simulink model "System_Design_Quadrocopter"  (Simulink 7.4)
settings: Solver=ode45  StartTime=0.0  StopTime=10.0  RelTol=1e-3
settings Model: Creator=roczit00  LastModifiedBy=roczit00

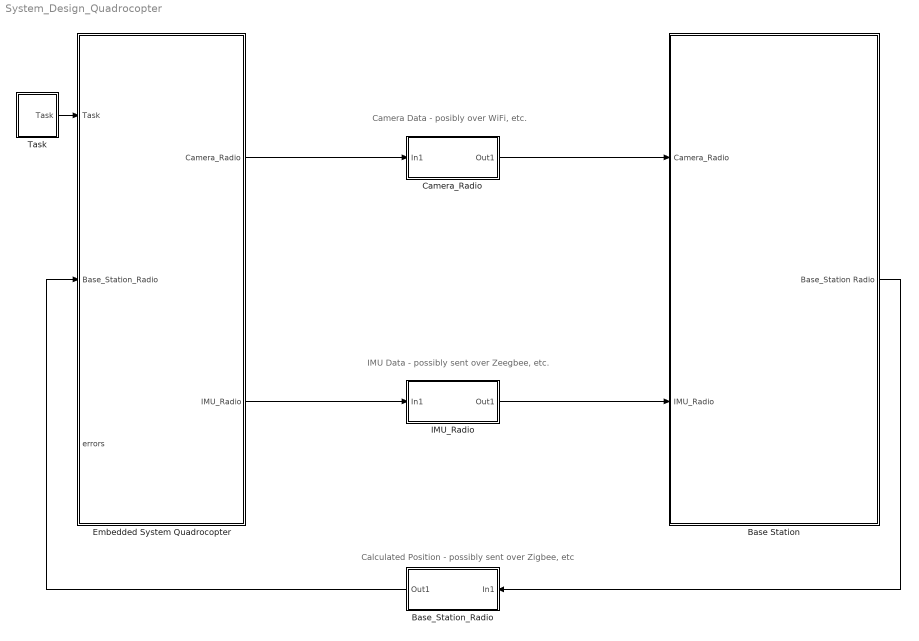
== system System_Design_Quadrocopter ==
  note: IMU Data - possibly sent over Zeegbee, etc.
  note: Calculated Position - possibly sent over Zigbee, etc
  note: Camera Data - posibly over WiFi, etc.
  Base Station : Subsystem
  Base_Station_Radio : Subsystem
  Camera_Radio : Subsystem
  Embedded System Quadrocopter : Subsystem
  IMU_Radio : Subsystem
  Task : Subsystem
  wires:
  Embedded System Quadrocopter/1(Camera_Radio) -> Camera_Radio/1(In1)
  Base Station/1(Base_Station Radio) -> Base_Station_Radio/1(In1)
  Base_Station_Radio/1(Out1) -> Embedded System Quadrocopter/2(Base_Station_Radio)
  Embedded System Quadrocopter/2(IMU_Radio) -> IMU_Radio/1(In1)
  IMU_Radio/1(Out1) -> Base Station/2(IMU_Radio)
  Camera_Radio/1(Out1) -> Base Station/1(Camera_Radio)
  Task/1(Task) -> Embedded System Quadrocopter/1(Task)

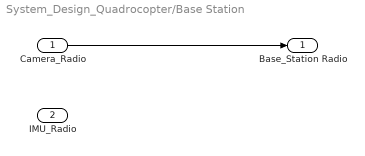
== system System_Design_Quadrocopter/Base Station ==
  Camera_Radio : Inport  OutDataType=fixdt(1, 16)  OutScaling=2^0
  IMU_Radio : Inport  Port=2  OutDataType=fixdt(1, 16)  OutScaling=2^0
  Base_Station Radio : Outport  OutDataType=fixdt(1, 16)  OutScaling=2^0
  wires:
  Camera_Radio/1 -> Base_Station Radio/1

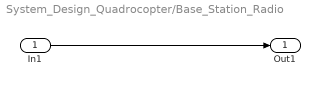
== system System_Design_Quadrocopter/Base_Station_Radio ==
  In1 : Inport  OutDataType=fixdt(1, 16)  OutScaling=2^0
  Out1 : Outport  OutDataType=fixdt(1, 16)  OutScaling=2^0
  wires:
  In1/1 -> Out1/1

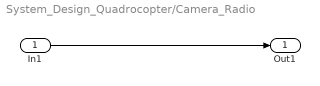
== system System_Design_Quadrocopter/Camera_Radio ==
  In1 : Inport  OutDataType=fixdt(1, 16)  OutScaling=2^0
  Out1 : Outport  OutDataType=fixdt(1, 16)  OutScaling=2^0
  wires:
  In1/1 -> Out1/1

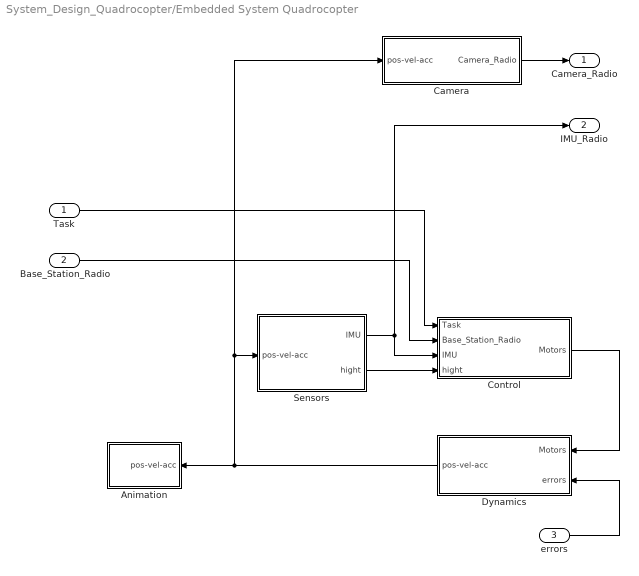
== system System_Design_Quadrocopter/Embedded System Quadrocopter ==
  Task : Inport  OutDataType=fixdt(1, 16)  OutScaling=2^0
  Base_Station_Radio : Inport  Port=2  OutDataType=fixdt(1, 16)  OutScaling=2^0
  errors : Inport  Port=3  OutDataType=fixdt(1, 16)  OutScaling=2^0
  Animation : Subsystem
  Camera : Subsystem
  Control : Subsystem
  Dynamics : Subsystem
  Sensors : Subsystem
  Camera_Radio : Outport  OutDataType=fixdt(1, 16)  OutScaling=2^0
  IMU_Radio : Outport  Port=2  OutDataType=fixdt(1, 16)  OutScaling=2^0
  wires:
  Sensors/1(IMU) -> Control/3(IMU), IMU_Radio/1
  Sensors/2(hight) -> Control/4(hight)
  errors/1 -> Dynamics/2(errors)
  Control/1(Motors) -> Dynamics/1(Motors)
  Dynamics/1(pos-vel-acc) -> Animation/1(pos-vel-acc), Sensors/1(pos-vel-acc), Camera/1(pos-vel-acc)
  Camera/1(Camera_Radio) -> Camera_Radio/1
  Base_Station_Radio/1 -> Control/2(Base_Station_Radio)
  Task/1 -> Control/1(Task)

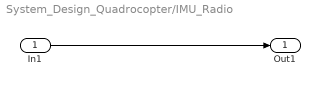
== system System_Design_Quadrocopter/IMU_Radio ==
  In1 : Inport  OutDataType=fixdt(1, 16)  OutScaling=2^0
  Out1 : Outport  OutDataType=fixdt(1, 16)  OutScaling=2^0
  wires:
  In1/1 -> Out1/1

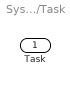
== system System_Design_Quadrocopter/Task ==
  Task : Outport  OutDataType=fixdt(1, 16)  OutScaling=2^0

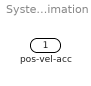
== system System_Design_Quadrocopter/Embedded System Quadrocopter/Animation ==
  pos-vel-acc : Inport  OutDataType=fixdt(1, 16)  OutScaling=2^0

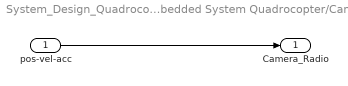
== system System_Design_Quadrocopter/Embedded System Quadrocopter/Camera ==
  pos-vel-acc : Inport  OutDataType=fixdt(1, 16)  OutScaling=2^0
  Camera_Radio : Outport  OutDataType=fixdt(1, 16)  OutScaling=2^0
  wires:
  pos-vel-acc/1 -> Camera_Radio/1

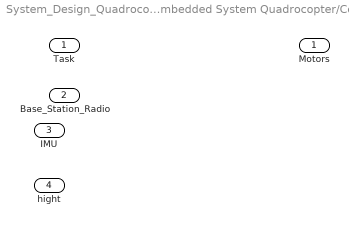
== system System_Design_Quadrocopter/Embedded System Quadrocopter/Control ==
  Task : Inport  OutDataType=fixdt(1, 16)  OutScaling=2^0
  Base_Station_Radio : Inport  Port=2  OutDataType=fixdt(1, 16)  OutScaling=2^0
  IMU : Inport  Port=3  OutDataType=fixdt(1, 16)  OutScaling=2^0
  hight : Inport  Port=4  OutDataType=fixdt(1, 16)  OutScaling=2^0
  Motors : Outport  OutDataType=fixdt(1, 16)  OutScaling=2^0

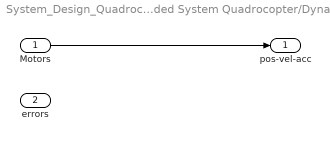
== system System_Design_Quadrocopter/Embedded System Quadrocopter/Dynamics ==
  Motors : Inport  OutDataType=fixdt(1, 16)  OutScaling=2^0
  errors : Inport  Port=2  OutDataType=fixdt(1, 16)  OutScaling=2^0
  pos-vel-acc : Outport  OutDataType=fixdt(1, 16)  OutScaling=2^0
  wires:
  Motors/1 -> pos-vel-acc/1

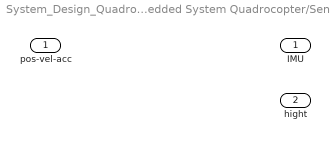
== system System_Design_Quadrocopter/Embedded System Quadrocopter/Sensors ==
  pos-vel-acc : Inport  OutDataType=fixdt(1, 16)  OutScaling=2^0
  IMU : Outport  OutDataType=fixdt(1, 16)  OutScaling=2^0
  hight : Outport  Port=2  OutDataType=fixdt(1, 16)  OutScaling=2^0
